simulink model "Phone_A"  (R2023a)
settings: Solver=FixedStepAuto  StartTime=0.0  StopTime=inf  RelTol=1e-3
undefined symbols (not defined in the file): Alert_Button, Angle_Fall_Detect, Boundary_Boolean, Boundary_Crossing_Check, DiscIntNeverNeededParam, Fall_Detection_Boolean, Horizontal_Speed, Latitude, Location_1, Location_2, Location_3, Longitude, Overspeed_Boolean, PhoneA
libraries: androiduilib x8, androidcommunicationlib x6, androidsensorlib x3, androidaudiovideolib x3
settings Model: Creator=patel  LastModifiedBy=patel
settings OptimizationCC: EnhancedBackFolding=on  PassReuseOutputArgsAs=Individual arguments  ZeroExternalMemoryAtStartup=off  ZeroInternalMemoryAtStartup=off  MaxStackSize=64  OptimizeBlockOrder=speed  DifferentSizesBufferReuse=on  OptimizationCustomize=off  EfficientTunableParamExpr=on
settings DebuggingCC: ParameterTunabilityLossMsg=error
settings HardwareCC: ProdBitPerPointer=32  ProdBitPerSizeT=32  ProdBitPerPtrDiffT=32  ProdLargestAtomicInteger=Long  ProdLargestAtomicFloat=Double  ProdWordSize=32  ProdHWDeviceType=ARM Compatible->ARM Cortex  UseEmbeddedCoderFeatures=off  UseSimulinkCoderFeatures=off
settings SFSimCC: MATLABDynamicMemAlloc=off
settings RTWCC: Description=Embedded Coder  SystemTargetFile=ert.tlc  HardwareBoard=Android Device  TLCOptions="-aInlineSetEventsForThisBaseRateFcn=TLC_FALSE -aSuppressMultiTaskScheduler=TLC_FALSE  -aRateBasedStepFcn=0"  TemplateMakefile=ert_default_tmf  RTWVerbose=off  Toolchain=Android SDK/NDK Tools
settings CodeAppCC: ForceParamTrailComments=on  IgnoreCustomStorageClasses=off  OperatorAnnotations=on  SimulinkDataObjDesc=on  SFDataObjDesc=on  InsertBlockDesc=on
settings ERTTargetCC: SupportNonInlinedSFcns=on

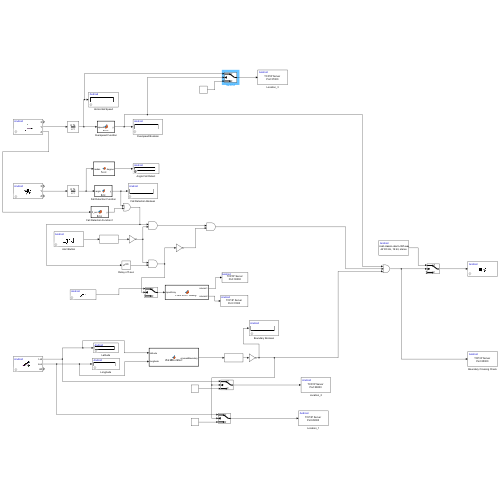
[thumbnail: Simulink's stored preview of the top-level diagram]
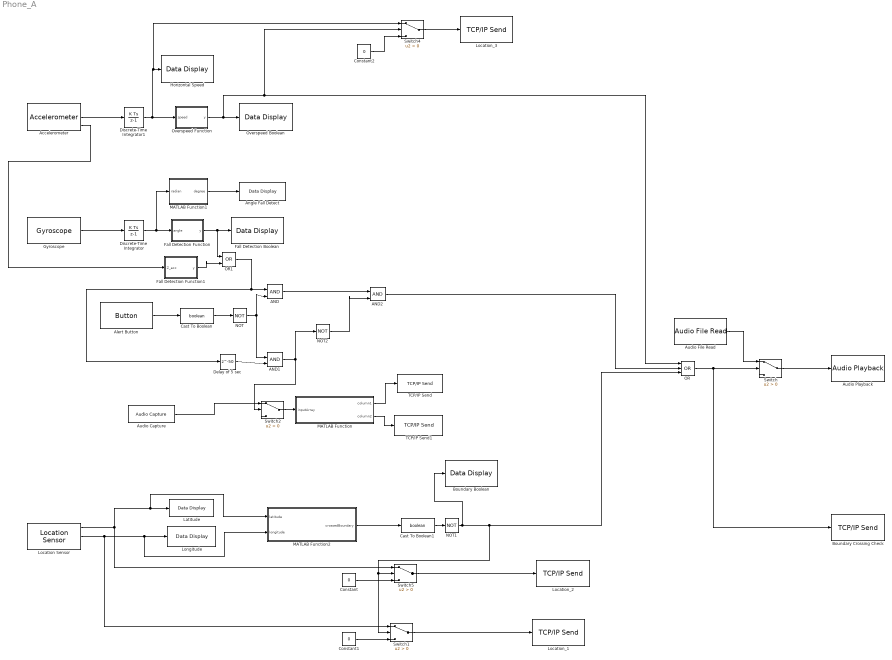
== system Phone_A ==
  AND : Logic  IconShape=distinctive  AllPortsSameDT=off  OutDataTypeStr=boolean
  AND1 : Logic  IconShape=distinctive  AllPortsSameDT=off  OutDataTypeStr=boolean
  AND2 : Logic  IconShape=distinctive  AllPortsSameDT=off  OutDataTypeStr=boolean
  Accelerometer : androidsensorlib/Accelerometer  OutputVector=off  SampleTime=0.1  BlockPlatform=Android
  Alert Button : androiduilib/Button  ButtonState=Not pressed  ButtonId=PhoneA/Alert_Button  State=off  SampleTime=0.1  BlockPlatform=Android
  Angle Fall Detect : androiduilib/Data Display  DataDisplayId=PhoneA/Angle_Fall_Detect  Format=Float  Precision=6  SimulateUsing=Code generation  blockPlatform=Android
  Audio Capture : androidaudiovideolib/Audio Capture  SampleFreq=44100  FrameSize=4410  SampleTime=0.1  SimulateUsing=Code generation  DeviceStr=0  QueueDuration=0  BlockPlatform=Android  AudioSamplingFreq=44100
  Audio File Read : androidaudiovideolib/Audio File Read  FileName=C:\Users\patel\Downloads\mixkit-classic-alarm-995.wav  FrameSize=4410
  Audio Playback : androidaudiovideolib/Audio Playback  SampleFreq=44100  AudioSamplingFreq=44100  SampleTime=0.1  DeviceStr=0  QueueDuration=0  BlockPlatform=Android
  Boundary Boolean : androiduilib/Data Display  DataDisplayId=PhoneA/Boundary_Boolean  Format=Float  Precision=6  SimulateUsing=Code generation  blockPlatform=Android
  Boundary Crossing Check : androidcommunicationlib/TCP//IP Send  TCPSendId=PhoneA/Boundary_Crossing_Check  Mode_=Server  LocalServerPort_=25000  RemoteAddr_=127.0.0.1  RemoteServerPort_=25000  ClientPortBindingSelection_=off  ClientPortToBind_=35000  BlockingMode_=off  BlockTimeout_=0.1
  Cast To Boolean : DataTypeConversion  OutDataTypeStr=boolean  SaturateOnIntegerOverflow=off  RndMeth=Floor
  Cast To Boolean1 : DataTypeConversion  OutDataTypeStr=boolean  SaturateOnIntegerOverflow=off  RndMeth=Floor
  Constant : Constant  Value=0
  Constant1 : Constant  Value=0
  Constant2 : Constant  Value=0
  Delay of 5 sec : Delay  DelayLength=50
  Discrete-Time Integrator : DiscreteIntegrator  SampleTime=-1  ICPrevOutput=DiscIntNeverNeededParam  ICPrevScaledInput=DiscIntNeverNeededParam
  Discrete-Time Integrator1 : DiscreteIntegrator  SampleTime=-1  ICPrevOutput=DiscIntNeverNeededParam  ICPrevScaledInput=DiscIntNeverNeededParam
  Fall Detection Boolean : androiduilib/Data Display  DataDisplayId=PhoneA/Fall_Detection_Boolean  Format=Float  Precision=6  SimulateUsing=Code generation  blockPlatform=Android
  Fall Detection Function : MATLAB Function  TreatAsAtomicUnit=on
  Fall Detection Function1 : MATLAB Function  TreatAsAtomicUnit=on
  Gyroscope : androidsensorlib/Gyroscope  OutputVector=off  SampleTime=0.1  BlockPlatform=Android
  Horizontal Speed : androiduilib/Data Display  DataDisplayId=PhoneA/Horizontal_Speed  Format=Float  Precision=6  SimulateUsing=Code generation  blockPlatform=Android
  Latitude : androiduilib/Data Display  DataDisplayId=PhoneA/Latitude  Format=Float  Precision=6  SimulateUsing=Code generation  blockPlatform=Android
  Location Sensor : androidsensorlib/Location Sensor  OutputVector=off  SampleTime=0.1  BlockPlatform=Android
  Location_1 : androidcommunicationlib/TCP//IP Send  TCPSendId=PhoneA/Location_1  Mode_=Server  LocalServerPort_=29000  RemoteAddr_=127.0.0.1  RemoteServerPort_=25000  ClientPortBindingSelection_=off  ClientPortToBind_=35000  BlockingMode_=off  BlockTimeout_=0.1
  Location_2 : androidcommunicationlib/TCP//IP Send  TCPSendId=PhoneA/Location_2  Mode_=Server  LocalServerPort_=28000  RemoteAddr_=127.0.0.1  RemoteServerPort_=25000  ClientPortBindingSelection_=off  ClientPortToBind_=35000  BlockingMode_=off  BlockTimeout_=0.1
  Location_3 : androidcommunicationlib/TCP//IP Send  TCPSendId=PhoneA/Location_3  Mode_=Server  LocalServerPort_=37000  RemoteAddr_=127.0.0.1  RemoteServerPort_=25000  ClientPortBindingSelection_=off  ClientPortToBind_=35000  BlockingMode_=off  BlockTimeout_=0.1
  Longitude : androiduilib/Data Display  DataDisplayId=PhoneA/Longitude  Format=Float  Precision=6  SimulateUsing=Code generation  blockPlatform=Android
  MATLAB Function : MATLAB Function  TreatAsAtomicUnit=on
  MATLAB Function1 : MATLAB Function  TreatAsAtomicUnit=on
  MATLAB Function2 : MATLAB Function  TreatAsAtomicUnit=on
  NOT : Logic  Operator=NOT  IconShape=distinctive  AllPortsSameDT=off  OutDataTypeStr=boolean
  NOT1 : Logic  Operator=NOT  IconShape=distinctive  AllPortsSameDT=off  OutDataTypeStr=boolean
  NOT2 : Logic  Operator=NOT  IconShape=distinctive  AllPortsSameDT=off  OutDataTypeStr=boolean
  OR : Logic  Operator=OR  Inputs=3  IconShape=distinctive  AllPortsSameDT=off  OutDataTypeStr=boolean
  OR1 : Logic  Operator=OR  IconShape=distinctive  AllPortsSameDT=off  OutDataTypeStr=boolean
  Overspeed Boolean : androiduilib/Data Display  DataDisplayId=PhoneA/Overspeed_Boolean  Format=Float  Precision=6  SimulateUsing=Code generation  blockPlatform=Android
  Overspeed Function : MATLAB Function  TreatAsAtomicUnit=on
  Switch : Switch  Criteria=u2 > Threshold  OutDataTypeStr=int16  SaturateOnIntegerOverflow=off  InputSameDT=off
  Switch1 : Switch  Criteria=u2 > Threshold  SaturateOnIntegerOverflow=off  InputSameDT=off
  Switch2 : Switch  Criteria=u2 > Threshold  OutDataTypeStr=int16  SaturateOnIntegerOverflow=off  InputSameDT=off
  Switch4 : Switch  Criteria=u2 > Threshold  OutDataTypeStr=int16  SaturateOnIntegerOverflow=off  InputSameDT=off
  Switch5 : Switch  Criteria=u2 > Threshold  SaturateOnIntegerOverflow=off  InputSameDT=off
  TCP/IP Send : androidcommunicationlib/TCP//IP Send  TCPSendId=PhoneA/TCP//IP_Send  Mode_=Server  LocalServerPort_=30000  RemoteAddr_=127.0.0.1  RemoteServerPort_=25000  ClientPortBindingSelection_=off  ClientPortToBind_=35000  BlockingMode_=off  BlockTimeout_=0.1
  TCP/IP Send1 : androidcommunicationlib/TCP//IP Send  TCPSendId=PhoneA/TCP//IP_Send1  Mode_=Server  LocalServerPort_=31000  RemoteAddr_=127.0.0.1  RemoteServerPort_=25000  ClientPortBindingSelection_=off  ClientPortToBind_=35000  BlockingMode_=off  BlockTimeout_=0.1
  wires:
  Accelerometer/2 -> Discrete-Time Integrator1/1
  Audio File Read/1 -> Switch/1
  Switch/1 -> Audio Playback/1
  Gyroscope/2 -> Discrete-Time Integrator/1
  Discrete-Time Integrator/1 -> MATLAB Function1/1(radian), Fall Detection Function/1(angle)
  Fall Detection Function/1(y) -> OR1/1, Fall Detection Boolean/1
  Alert Button/1 -> Cast To Boolean/1
  Cast To Boolean/1 -> NOT/1
  NOT/1 -> AND1/1, AND/2
  Delay of 5 sec/1 -> AND1/2
  Location Sensor/1 -> Switch5/1, MATLAB Function2/1(latitude), Latitude/1
  Location Sensor/2 -> Switch1/1, MATLAB Function2/2(longitude), Longitude/1
  MATLAB Function1/1(degree) -> Angle Fall Detect/1
  MATLAB Function2/1(crossedBoundary) -> Cast To Boolean1/1
  Cast To Boolean1/1 -> NOT1/1
  Accelerometer/3 -> Fall Detection Function1/1(Z_acc)
  Fall Detection Function1/1(y) -> OR1/2
  OR1/1 -> Delay of 5 sec/1, AND/1
  AND1/1 -> NOT2/1, Switch2/2
  Audio Capture/1 -> Switch2/1
  Switch2/1 -> MATLAB Function/1(inputArray)
  MATLAB Function/1(column1) -> TCP/IP Send/1
  MATLAB Function/2(column2) -> TCP/IP Send1/1
  OR/1 -> Boundary Crossing Check/1, Switch/2
  AND/1 -> AND2/1
  AND2/1 -> OR/2
  NOT2/1 -> AND2/2
  Discrete-Time Integrator1/1 -> Overspeed Function/1(speed), Switch4/1, Horizontal Speed/1
  NOT1/1 -> Switch1/2, Switch5/2, OR/3, Boundary Boolean/1
  Overspeed Function/1(y) -> Switch4/2, OR/1, Overspeed Boolean/1
  Switch5/1 -> Location_2/1
  Switch1/1 -> Location_1/1
  Constant/1 -> Switch5/3
  Constant1/1 -> Switch1/3
  Constant2/1 -> Switch4/3
  Switch4/1 -> Location_3/1

== matlab function Phone_A/Fall Detection Function ==
  data: angle input; y output
function y = func(angle)

if (abs(angle) > 0.75) 
    y = true;
else
    y = false;
end
end

== matlab function Phone_A/MATLAB Function2 ==
  data: latitude input; crossedBoundary output; longitude input
function crossedBoundary = checkBoundary(latitude, longitude)
    % Check if the latitude and longitude are within the defined boundary

    %lat=[23.209492,23.210616,23.210635,23.209495];
    %long=[72.683352,72.683376,72.684304,72.684249];
    %Vadodara
    lat=[22.288605,22.288540,22.288533,22.288592];
    long=[73.122303,73.122310,73.122217,73.122205];
    %lat=[23.209844,23.209835,23.209652,23.209650];
    %long=[72.683674,72.684037,72.683987,72.683694];
    crossedBoundary = inpolygon(latitude, longitude, lat, long);
end

== matlab function Phone_A/Overspeed Function ==
  data: speed input; y output
function y = func(speed)

if (abs(speed) > 25) 
    y = true;
else
    y = false;
end
end

== matlab function Phone_A/Fall Detection Function1 ==
  data: Z_acc input; y output
function y = func(Z_acc)

if abs(Z_acc) < 0.5
    y = true;
else
    y = false;
end
end

== matlab function Phone_A/MATLAB Function ==
  data: inputArray input; column1 output; column2 output
function [column1, column2] = convertTo1DArrays(inputArray)
    % Check if inputArray is a valid Nx2 array
    [nRows, nCols] = size(inputArray);
    if nCols ~= 2
        error('Input must be an Nx2 array.');
    end

    % Extract the columns into separate 1D arrays
    column1 = inputArray(:, 1);
    column2 = inputArray(:, 2);
end

== matlab function Phone_A/MATLAB Function1 ==
  data: radian input; degree output
function degree = func(radian)
    degree = rad2deg(radian);
end
